simulink model "Copy_of_EmraxEfficiencySimulation"  (R2023b)
settings: Solver=VariableStepAuto  StartTime=0.0  StopTime=2862  MinStep=1e-6  RelTol=1e-3
model workspace (MAT data in the model file):
  surfaceBlockParameters = Simulink.LookupTable
  surfaceBlockParameters.Table = Simulink.lookuptable.Table
  surfaceBlockParameters.Table.Value = [0.86  0.86  0.86  0.86  0.86  0.86  0.86  0.86  0.86  0.86  0.86; 0.86  0.86  0.873462974516  0.88120855107  0.887257540982  0.881274655143  0.875257466166  0.861277049262  0.86  0.86  0.86; 0.86  0.869449686674  0.901077583035  0.940198386719  0.941242897487  0.93026047687  0.938338197526  0.920269194974  0.901654311136  0.876925457275  0.86; 0.86  0.871584749393  0.920465089637  0.946640854986  0.955098186441  0.959157998253  0.952414685218  0.944193761546  0.931829553709  0.909148651806  0.86; 0.86  0.873600000005  0.920099009905  0.957797916669  0.96  0.96  0.955048161402  0.948313069463  0.940179875207  0.910126940639  0.86; 0.86  0.873810561857  0.92068092196  0.957924221415  0.96  0.96  0.954746546712  0.948709551276  0.940686275533  0.907960706815  0.86; 0.86  0.870474457304  0.920710477493  0.954650751967  0.96  0.959091387712  0.953985871947  0.947696813236  0.940596870284  0.905794472991  0.86; 0.86  0.864180163786  0.915794053212  0.947295039135  0.96  0.957068912618  0.952635425118  0.946716594455  0.940428015723  0.903628239166  0.86; 0.86  0.86  0.881189733357  0.926126919259  0.949537413693  0.95356721004  0.95044514073  0.946547739895  0.940259161163  0.900401534397  0.86; 0.86  0.86  0.86  0.89019154205  0.934327668899  0.937067800236  0.945715791697  0.945163394756  0.940090306602  0.909654921019  0.86; 0.86  0.86  0.86  0.86  0.86  0.901026892928  0.936959816894  0.940077714286  0.939615450249  0.908828254349  0.86]
  surfaceBlockParameters.Table.Dimensions = [11 11]
  surfaceBlockParameters.Table.DataType = 'auto'
  surfaceBlockParameters.Table.FieldName = 'Table_Efficiency_Map_Efficiency'
  surfaceBlockParameters.Breakpoints(1) = Simulink.lookuptable.Breakpoint
  surfaceBlockParameters.Breakpoints(1).Value = [0 550 1100 1650 2200 2750 3300 3850 4400 4950 5500]
  surfaceBlockParameters.Breakpoints(1).TunableSizeName = 'N1'
  surfaceBlockParameters.Breakpoints(1).Dimensions = [1 11]
  surfaceBlockParameters.Breakpoints(1).DataType = 'auto'
  surfaceBlockParameters.Breakpoints(1).FieldName = 'BP1_Efficiency_Map_RPM'
  surfaceBlockParameters.Breakpoints(2) = Simulink.lookuptable.Breakpoint
  surfaceBlockParameters.Breakpoints(2).Value = [0 25 50 75 100 125 150 175 200 225 250]
  surfaceBlockParameters.Breakpoints(2).TunableSizeName = 'N2'
  surfaceBlockParameters.Breakpoints(2).Dimensions = [1 11]
  surfaceBlockParameters.Breakpoints(2).DataType = 'auto'
  surfaceBlockParameters.Breakpoints(2).FieldName = 'BP2_Efficiency_Map_Torque'
  surfaceBlockParameters.AllowMultipleInstancesOfTypeToHaveDifferentTableBreakpointSizes = 0
  surfaceBlockParameters.SupportTunableSize = 0
  surfaceBlockParameters.StructTypeInfo = Simulink.lookuptable.StructTypeInfo
  surfaceBlockParameters.StructTypeInfo.Name = 'surfaceBlockParameters_type'
  surfaceBlockParameters.StructTypeInfo.DataScope = 'Auto'
values from neighbouring files (symbols this model uses):
  battery = {}    [init_file.m]
  motor = {}    [init_file.m]
  powertrain = {}    [init_file.m]
libraries: nesl_utility x7, fl_lib x6, batteryecm_lib x1, spsFirstOrderFilterLib x1, mcbcontrolslib x1
settings Model: SimulationMode=accelerator  Creator=benli  LastModifiedBy=benli
settings SolverCC: MaxConsecutiveMinStep=10

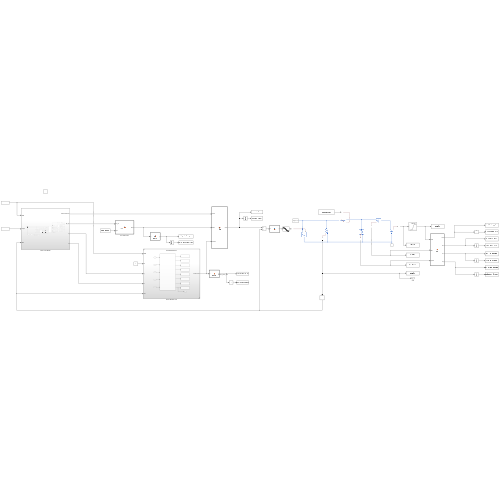
[thumbnail: Simulink's stored preview of the top-level diagram]
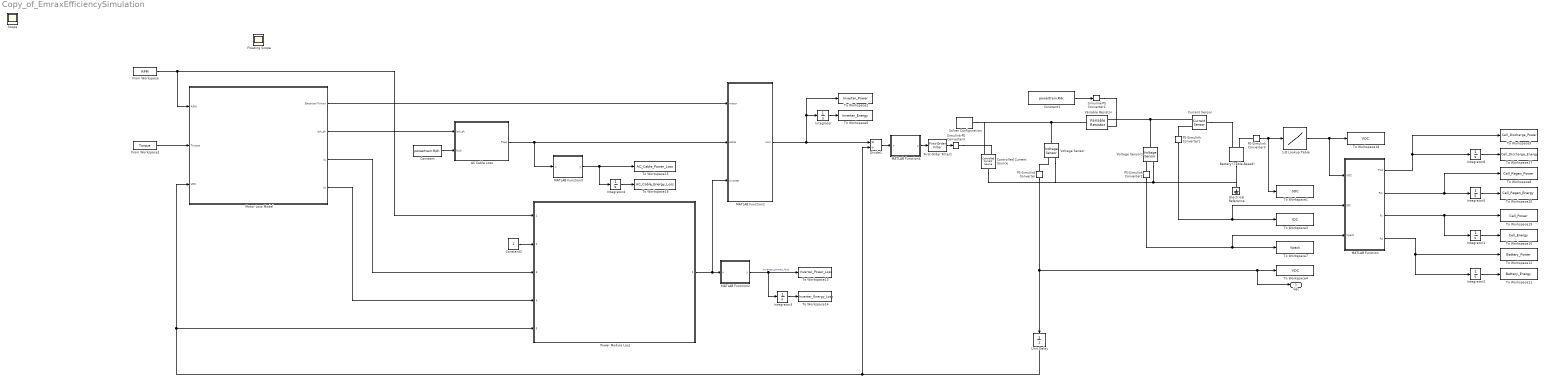
== system Copy_of_EmraxEfficiencySimulation ==
  1-D Lookup Table : Lookup_n-D  NumberOfTableDimensions=1  BreakpointsForDimension1=battery.soc_x_ocv_y(:,1)  Table=battery.soc_x_ocv_y(:,2)*battery.S  InternalRulePriority=Speed  RndMeth=Simplest
  AC Cable Loss : MATLAB Function  TreatAsAtomicUnit=on
  Battery (Table-Based) : batteryecm_lib/Battery (Table-Based)  SOC_vec=battery.soc_x_ocv_y(:,1)  T_dependence=simscape.enum.tablebattery.temperature_dependence.no  prm_dir=simscape.enum.tablebattery.prm_dir.noCurrentDirectionality  T_vec=[278, 293, 313] K  V0_mat=[3.49, 3.5, 3.51; 3.55, 3.57, 3.56; 3.62, 3.63, 3.64; 3.71, 3.71, 3.72; 3.91, 3.93, 3.94; 4.07, 4.08, 4.08; 4.19, 4.19, 4.19] V  V0_vec=battery.soc_x_ocv_y(:,2)*battery.S V  V_range=[0, 700] V  R0_mat=[.0117, .0085, .009; .011, .0085, .009; .0114, .0087, .0092; .0107, .0082, .0088; .0107, .0083, .0091; .0113, .0085, .0089; .0116, .0085, .0089] Ohm  R0_vec=battery.Rdc*ones(1002,1) Ohm  R0_dis_mat=[.0117, .0085, .009; .011, .0085, .009; .0114, .0087, .0092; .0107, .0082, .0088; .0107, .0083, .0091; .0113, .0085, .0089; .0116, .0085, .0089] Ohm  R0_dis_vec=[.0085, .0085, .0087, .0082, .0083, .0085, .0085] Ohm  R0_ch_mat=[.0117, .0085, .009; .011, .0085, .009; .0114, .0087, .0092; .0107, .0082, .0088; .0107, .0083, .0091; .0113, .0085, .0089; .0116, .0085, .0089] Ohm  R0_ch_vec=[.0085, .0085, .0087, .0082, .0083, .0085, .0085] Ohm  AH=battery.Ah*battery.P A*hr  prm_leak=simscape.enum.tablebattery.prm_leak.disabled  Rleak_vec=[8000, 7000, 6000] Ohm  Rleak=7e3 Ohm  extrapolation_option=simscape.enum.extrapolation.linear  SOC_port=simscape.enum.tablebattery.enable.yes  prm_dyn=simscape.enum.tablebattery.prm_dyn.off  R1_mat=[.0109, .0029, .0013; .0069, .0024, .0012; .0047, .0026, .0013; .0034, .0016, .001; .0033, .0023, .0014; .0033, .0018, .0011; .0028, .0017, .0011] Ohm  R1_vec=[.0029, .0024, .0026, .0016, .0023, .0018, .0017] Ohm  tau1_mat=[20, 36, 39; 31, 45, 39; 109, 105, 61; 36, 29, 26; 59, 77, 67; 40, 33, 29; 25, 39, 33] s  tau1_vec=[36, 45, 105, 29, 77, 33, 39] s  R2_mat=[.0109, .0029, .0013; .0069, .0024, .0012; .0047, .0026, .0013; .0034, .0016, .001; .0033, .0023, .0014; .0033, .0018, .0011; .0028, .0017, .0011] Ohm  R2_vec=[.0029, .0024, .0026, .0016, .0023, .0018, .0017] Ohm  tau2_mat=[20, 36, 39; 31, 45, 39; 109, 105, 61; 36, 29, 26; 59, 77, 67; 40, 33, 29; 25, 39, 33] s  tau2_vec=[36, 45, 105, 29, 77, 33, 39] s  R3_mat=[.0109, .0029, .0013; .0069, .0024, .0012; .0047, .0026, .0013; .0034, .0016, .001; .0033, .0023, .0014; .0033, .0018, .0011; .0028, .0017, .0011] Ohm  R3_vec=[.0029, .0024, .0026, .0016, .0023, .0018, .0017] Ohm  tau3_mat=[20, 36, 39; 31, 45, 39; 109, 105, 61; 36, 29, 26; 59, 77, 67; 40, 33, 29; 25, 39, 33] s  tau3_vec=[36, 45, 105, 29, 77, 33, 39] s  R4_mat=[.0109, .0029, .0013; .0069, .0024, .0012; .0047, .0026, .0013; .0034, .0016, .001; .0033, .0023, .0014; .0033, .0018, .0011; .0028, .0017, .0011] Ohm  R4_vec=[.0029, .0024, .0026, .0016, .0023, .0018, .0017] Ohm  tau4_mat=[20, 36, 39; 31, 45, 39; 109, 105, 61; 36, 29, 26; 59, 77, 67; 40, 33, 29; 25, 39, 33] s  tau4_vec=[36, 45, 105, 29, 77, 33, 39] s  R5_mat=[.0109, .0029, .0013; .0069, .0024, .0012; .0047, .0026, .0013; .0034, .0016, .001; .0033, .0023, .0014; .0033, .0018, .0011; .0028, .0017, .0011] Ohm  R5_vec=[.0029, .0024, .0026, .0016, .0023, .0018, .0017] Ohm  tau5_mat=[20, 36, 39; 31, 45, 39; 109, 105, 61; 36, 29, 26; 59, 77, 67; 40, 33, 29; 25, 39, 33] s  tau5_vec=[36, 45, 105, 29, 77, 33, 39] s  prm_fade=simscape.enum.tablebattery.prm_fade.disabled  N0=100  dV0=0  dR0=0  dAH=0  dRleak=0  dR1=0  dR2=0  dR3=0  dR4=0  dR5=0  N0vec=[0, 100, 200, 300]  Tfadevec=[298.15, 323.15] K  dV0vec=[0, 0, 0, 0]  dR0vec=[0, 0, 0, 0]  dAHvec=[0, 0, 0, 0]  dRleakvec=[0, 0, 0, 0]  dR1vec=[0, 0, 0, 0]  dR2vec=[0, 0, 0, 0]  dR3vec=[0, 0, 0, 0]  dR4vec=[0, 0, 0, 0]  dR5vec=[0, 0, 0, 0]  dV0mat=[0, 0; 0, 0; 0, 0; 0, 0]  dR0mat=[0, 0; 0, 0; 0, 0; 0, 0]  dAHmat=[0, 0; 0, 0; 0, 0; 0, 0]  dRleakmat=[0, 0; 0, 0; 0, 0; 0, 0]  dR1mat=[0, 0; 0, 0; 0, 0; 0, 0]  dR2mat=[0, 0; 0, 0; 0, 0; 0, 0]  dR3mat=[0, 0; 0, 0; 0, 0; 0, 0]  dR4mat=[0, 0; 0, 0; 0, 0; 0, 0]  dR5mat=[0, 0; 0, 0; 0, 0; 0, 0]  prm_age_modeling=simscape.enum.tablebattery.prm_age_modeling.equation  storage_dt_age_vec=[0] d  storage_T_age_vec=[273] K  prm_age_OCV=simscape.enum.tablebattery.prm_age_OCV.OCV  OCV_age=0.9  SOC_age=0.6  prm_age_resistance=simscape.enum.tablebattery.prm_age.disabled  OCV_scaling_age_resistance=2.2134e6  OCV_offset_age_resistance=1.632e6  temp_exp_age_resistance=0.515833569 V  t_exp_age_resistance=0.75  T_age_vec_resistance=[273.15, 298.15, 323.15] K  dt_age_vec_resistance=[0, 90, 180, 270] d  dR0_age_vec=[0, 0, 0]  t_meas_dR0_age=100 d  dR0_age_mat=[0, 0, 0; 0, 0, 0; 0, 0, 0; 0, 0, 0]  prm_age_capacity=simscape.enum.tablebattery.prm_age.disabled  OCV_scaling_age_capacity=1.5097e07  OCV_offset_age_capacity=8.3625e06  temp_exp_age_capacity=0.6011 V  t_exp_age_capacity=0.75  T_age_vec_capacity=[273.15, 298.15, 323.15] K  dt_age_vec_capacity=[0, 90, 180, 270] d  dAH_age_vec=[0, 0, 0]  t_meas_dAH_age=100 d  dAH_age_mat=[0, 0, 0; 0, 0, 0; 0, 0, 0; 0, 0, 0]  thermal_port=simscape.enum.thermaleffects.omit  temperature=298.15 K  thermal_mass=100 J/K  i_specify=off  i_priority=None  i=0 A  i_nominal_specify=off  i_nominal_unit=A  i_nominal_value=1  v_specify=off  v_priority=None  v=0 V  v_nominal_specify=off  v_nominal_unit=V  v_nominal_value=1  stateOfCharge_specify=on  stateOfCharge_priority=High  stateOfCharge=0.938  stateOfCharge_nominal_specify=off  stateOfCharge_nominal_unit=1  stateOfCharge_nominal_value=0.95  num_cycles_specify=off  num_cycles_priority=High  num_cycles=0  num_cycles_nominal_specify=off  num_cycles_nominal_unit=1  num_cycles_nominal_value=1  cell_temperature_specify=off  cell_temperature_priority=High  cell_temperature=298.15 K  cell_temperature_nominal_specify=off  cell_temperature_nominal_unit=K  cell_temperature_nominal_value=1
      settings: InternalSimscapePortConfiguration="{\"Bottom\":[],\"Left\":[{\"id\":\"p\",\"label\":\"+\",\"type\":\"foundation.electrical.electrical\"},{\"id\":\"soc\",\"label\":\"SOC\",\"type\":\"output\"}],\"Right\":[{\"id\":\"n\",\"label\":\"-\",\"type\":\"foundation.electrical.electrical\"}],\"Top\":[]}"
      settings: LibrarySourceBlock=|
      | batt_lib/Cells/Battery
      | (Table-Based)
  Constant : Constant  Value=powertrain.Rph
  Constant1 : Constant  Value=powertrain.Rdc
  Constant2 : Constant
  Controlled Current Source : fl_lib/Electrical/Electrical Sources/Controlled Current Source
  Current Sensor : fl_lib/Electrical/Electrical Sensors/Current Sensor
  Divide1 : Product  Inputs=*/
  Electrical Reference : fl_lib/Electrical/Electrical Elements/Electrical Reference
  First-Order Filter1 : spsFirstOrderFilterLib/First-Order Filter  FilterType=Lowpass  Tc=5e-2  Ts=0  Initialize=on  Vac_Init=[0, 0, 60]  Vdc_Init=0  PlotResponse=off  FreqRange="[0,  200,  1]"
  Floating Scope : Scope
      settings: Floating=on
  From Workspace : FromWorkspace  VariableName=RPM  SampleTime=0.05
  From Workspace1 : FromWorkspace  VariableName=Torque  SampleTime=0.05
  Integrator{,1..6} (7 alike) : Integrator
  MATLAB Function : MATLAB Function  TreatAsAtomicUnit=on
  MATLAB Function1 : MATLAB Function  TreatAsAtomicUnit=on
  MATLAB Function2 : MATLAB Function  TreatAsAtomicUnit=on
  MATLAB Function3 : MATLAB Function  TreatAsAtomicUnit=on
  MATLAB Function4 : MATLAB Function  TreatAsAtomicUnit=on
  Motor Loss Model : Subsystem
  PS-Simulink Converter{,1..3} (4 alike) : nesl_utility/PS-Simulink Converter  PhysicalDomain=network_engine_domain  SubClassName=ps_output  LeftPortType=input  RightPortType=output  PseudoPeriodic=off  Frequencies=[]  VectorFormat=inherit  Unit=inherit  AffineConversion=off
  Power Module Loss : Subsystem  ReferencedSubsystem=PowerModuleLoss
  Simulink-PS Converter2 : nesl_utility/Simulink-PS Converter  PhysicalDomain=network_engine_domain  SubClassName=ps_input  LeftPortType=input  RightPortType=output  PseudoPeriodic=off  Frequencies=[]  NoiseDistribution=none  NoiseParameters=[]  Unit=1  AffineConversion=off  FilteringAndDerivatives=provide  SimscapeFilterOrder=1  InputFilterTimeConstant=0.001  UdotUserProvided=0
  Simulink-PS Converter3 : nesl_utility/Simulink-PS Converter  PhysicalDomain=network_engine_domain  SubClassName=ps_input  LeftPortType=input  RightPortType=output  PseudoPeriodic=off  Frequencies=[]  NoiseDistribution=none  NoiseParameters=[]  Unit=1  AffineConversion=off  FilteringAndDerivatives=provide  SimscapeFilterOrder=1  InputFilterTimeConstant=0.001  UdotUserProvided=0
  Solver Configuration : nesl_utility/Solver Configuration  PhysicalDomain=network_engine_domain  SubClassName=solver  LeftPortType=input  RightPortType=generic  Tones=[]  Harmonics=[]  SimulateNoise=off  Profile=off  UseLocalSampling=off  EnableSwitchedLinearOptims=on  FrequencyDomain=off  UseCCode=off  RelTol=0.001  AbsTol=0.001  MinStep=1e-09  ToWorkspace=off  RevertToSquareIcSolve=off  NumHomotopyIterations=100  PhasorMode=off  PhasorModeNumHarmonics=1  ConsistencySolver=NEWTON_XTOL_AFTER_FTOL  IndexReductionMethod=DerivativeReplacement  DoDC=off  ResidualTolerance=1e-09  ConsistencyTolSource=GLOBAL  ConsistencyAbsTol=0.01  ConsistencyRelTol=0.01  ConsistencyTolFactor=0.001  UseLocalSolver=off  LocalSolverChoice=NE_PARTITIONING_ADVANCER  ResolveIndetEquations=on  FunctionEvalNumThread=1  LocalSolverSampleTime=0.0001  DoFixedCost=off  MaxNonlinIter=3  MaxModeIter=2  ComputeImpulses=off  ImpulseIterations=2  LinearAlgebra=auto  LinearAlgebraNumThread=0  EquationFormulation=NE_TIME_EF  DelaysMemoryBudget=1024  AutomaticFiltering=on  FilteringTimeConstant=0.001  PartitionStorageMethod=AS_NEEDED  PartitionMemoryBudget=1024  PartitionMethod=ROBUST  MultibodyUseLocalSolver=off  MultibodyLocalSolverChoice=ODE1  MultibodyLocalSolverSampleTime=0.001
  To Workspace1 : ToWorkspace  VariableName=SOC  SampleTime=-1
  To Workspace10 : ToWorkspace  VariableName=Cell_Energy  SampleTime=-1
  To Workspace11 : ToWorkspace  VariableName=Battery_Energy  SampleTime=-1
  To Workspace12 : ToWorkspace  VariableName=Battery_Power  SampleTime=-1
  To Workspace13 : ToWorkspace  VariableName=Inverter_Power_Loss  SampleTime=-1
  To Workspace14 : ToWorkspace  VariableName=Inverter_Energy_Loss  SampleTime=-1
  To Workspace15 : ToWorkspace  VariableName=AC_Cable_Power_Loss  SampleTime=-1
  To Workspace16 : ToWorkspace  VariableName=AC_Cable_Energy_Loss  SampleTime=-1
  To Workspace17 : ToWorkspace  VariableName=Cell_Discharge_Energy  SampleTime=-1
  To Workspace18 : ToWorkspace  VariableName=VOC  SampleTime=-1
  To Workspace19 : ToWorkspace  VariableName=Cell_Power  SampleTime=-1
  To Workspace2 : ToWorkspace  VariableName=Inverter_Power  SampleTime=-1
  To Workspace20 : ToWorkspace  VariableName=Cell_Regen_Energy  SampleTime=-1
  To Workspace3 : ToWorkspace  VariableName=IDC  SampleTime=-1
  To Workspace4 : ToWorkspace  VariableName=VDC  SampleTime=-1
  To Workspace6 : ToWorkspace  VariableName=Inverter_Energy  SampleTime=-1
  To Workspace7 : ToWorkspace  VariableName=Vpack  SampleTime=-1
  To Workspace8 : ToWorkspace  VariableName=Cell_Regen_Power  SampleTime=-1
  To Workspace9 : ToWorkspace  VariableName=Cell_Discharge_Power  SampleTime=-1
  Unit Delay : UnitDelay  InitialCondition=battery.Voc  SampleTime=-1  HasFrameUpgradeWarning=on
  Variable Resistor : fl_lib/Electrical/Electrical Elements/Variable Resistor  Rmin=1 mOhm  thermalEnable=false  thermal_mass=1 J/K  i_specify=off  i_priority=None  i=0 A  i_nominal_specify=off  i_nominal_unit=A  i_nominal_value=1  v_specify=off  v_priority=None  v=0 V  v_nominal_specify=off  v_nominal_unit=V  v_nominal_value=1  T_specify=off  T_priority=None  T=300 K  T_nominal_specify=off  T_nominal_unit=K  T_nominal_value=1
  Voltage Sensor : fl_lib/Electrical/Electrical Sensors/Voltage Sensor
  Voltage Sensor1 : fl_lib/Electrical/Electrical Sensors/Voltage Sensor
  Vdc : Outport
  Scope : Scope
  wires:
  Constant/1 -> AC Cable Loss/2(Rph)
  Integrator3/1 -> To Workspace14/1
  Power Module Loss/1 -> MATLAB Function1/3(inverter), MATLAB Function2/1(u)
  Motor Loss Model/2(Iph_pk) -> AC Cable Loss/1(Iph_pk)
  From Workspace/1 -> Motor Loss Model/1(RPM), Power Module Loss/1
  MATLAB Function1/1(sum) -> Divide1/1, To Workspace2/1, Integrator/1
  PS-Simulink Converter3/1 -> To Workspace1/1, 1-D Lookup Table/1
  Motor Loss Model/3(Iq) -> Power Module Loss/3
  Unit Delay/1 -> Motor Loss Model/3(VDC), Power Module Loss/5, Divide1/2
  Constant1/1 -> Simulink-PS Converter2/1
  From Workspace1/1 -> Motor Loss Model/2(Torque)
  Motor Loss Model/4(Id) -> Power Module Loss/4
  Motor Loss Model/1(Electrical Power) -> MATLAB Function1/1(motor)
  PS-Simulink Converter1/1 -> To Workspace3/1, MATLAB Function/2(IDC)
  Integrator2/1 -> To Workspace11/1
  Integrator1/1 -> To Workspace10/1
  MATLAB Function3/1(y) -> To Workspace15/1, Integrator4/1
  AC Cable Loss/1(PLac) -> MATLAB Function3/1(u), MATLAB Function1/2(cable)
  Integrator6/1 -> To Workspace17/1
  Constant2/1 -> Power Module Loss/2
  Integrator/1 -> To Workspace6/1
  First-Order Filter1/1 -> Simulink-PS Converter3/1
  Integrator4/1 -> To Workspace16/1
  MATLAB Function/3(Pc) -> To Workspace19/1, Integrator1/1
  MATLAB Function4/1(y) -> First-Order Filter1/1
  1-D Lookup Table/1 -> To Workspace18/1, MATLAB Function/1(VOC)
  MATLAB Function/4(Pp) -> To Workspace12/1, Integrator2/1
  MATLAB Function/2(Pcr) -> To Workspace8/1, Integrator5/1
  MATLAB Function2/1(y) -> To Workspace13/1, Integrator3/1  "inverter_power_loss"
  Integrator5/1 -> To Workspace20/1
  PS-Simulink Converter/1 -> Unit Delay/1, Vdc/1, To Workspace4/1
  PS-Simulink Converter2/1 -> To Workspace7/1, MATLAB Function/3(Vpack)
  MATLAB Function/1(Pcd) -> Integrator6/1, To Workspace9/1
  Divide1/1 -> MATLAB Function4/1(u)
  connections:
  Voltage Sensor1/RConn2 -- Voltage Sensor/RConn2 -- Controlled Current Source/LConn1 -- Battery (Table-Based)/RConn1 -- Electrical Reference/LConn1
  Current Sensor/RConn2 -- Voltage Sensor1/LConn1 -- Variable Resistor/LConn2
  Voltage Sensor/LConn1 -- Controlled Current Source/RConn2 -- Solver Configuration/RConn1 -- Variable Resistor/RConn1
  PS-Simulink Converter3/LConn1 -- Battery (Table-Based)/LConn2
  Current Sensor/LConn1 -- Battery (Table-Based)/LConn1
  Simulink-PS Converter3/RConn1 -- Controlled Current Source/RConn1
  Current Sensor/RConn1 -- PS-Simulink Converter1/LConn1
  Simulink-PS Converter2/RConn1 -- Variable Resistor/LConn1
  PS-Simulink Converter/LConn1 -- Voltage Sensor/RConn1
  PS-Simulink Converter2/LConn1 -- Voltage Sensor1/RConn1

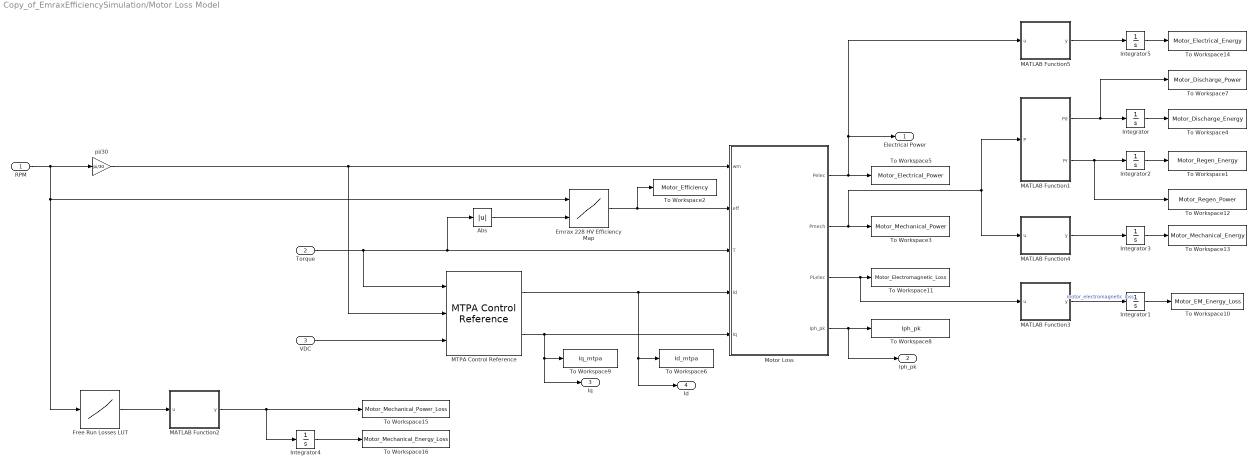
== system Copy_of_EmraxEfficiencySimulation/Motor Loss Model ==
  RPM : Inport
  Torque : Inport  Port=2
  VDC : Inport  Port=3
  Abs : Abs  SaturateOnIntegerOverflow=off
  Emrax 228 HV Efficiency Map : Lookup_n-D  DataSpecification=Lookup table object  LookupTableObject=surfaceBlockParameters  BreakpointsForDimension1=[1:3]  BreakpointsForDimension2=[1:3]  ExtrapMethod=Clip  InternalRulePriority=Speed  RndMeth=Simplest
      settings: AttributesFormatString=Extrapolation=%<ExtrapMethod>  InputPortMap=u0,u1
  Free Run Losses LUT : Lookup_n-D  NumberOfTableDimensions=1  BreakpointsForDimension1=motor.RPM_x_Power_y(:, 1)  Table=motor.RPM_x_Power_y(:, 2)  InternalRulePriority=Speed  RndMeth=Simplest
  Integrator{,1..5} (6 alike) : Integrator
  MATLAB Function1 : MATLAB Function  TreatAsAtomicUnit=on
  MATLAB Function2 : MATLAB Function  TreatAsAtomicUnit=on
  MATLAB Function3 : MATLAB Function  TreatAsAtomicUnit=on
  MATLAB Function4 : MATLAB Function  TreatAsAtomicUnit=on
  MATLAB Function5 : MATLAB Function  TreatAsAtomicUnit=on
  MTPA Control Reference : mcbcontrolslib/MTPA Control Reference  VariantSelect=Interior PMSM  polePairs=motor.Pp  Rs=motor.Rw  Ld=motor.Ld  Lq=motor.Lq  FluxPM=motor.Lambda_m  ilimit=motor.I_lim  Vdc_input_select=Input port  V_dc=500  Units=SI Units  N_base=4107  I_base=19.3  T_base=1  V_base=24/sqrt(3)  N_base_disp=3182  MTPAiterator=on  iterCount=10
      settings: LibrarySourceBlock=mcblib/Controls/Control Reference/MTPA Control Reference
  Motor Loss : MATLAB Function  TreatAsAtomicUnit=on
  To Workspace1 : ToWorkspace  VariableName=Motor_Regen_Energy  SampleTime=-1
  To Workspace10 : ToWorkspace  VariableName=Motor_EM_Energy_Loss  SampleTime=-1
  To Workspace11 : ToWorkspace  VariableName=Motor_Electromagnetic_Loss  SampleTime=-1
  To Workspace12 : ToWorkspace  VariableName=Motor_Regen_Power  SampleTime=-1
  To Workspace13 : ToWorkspace  VariableName=Motor_Mechanical_Energy  SampleTime=-1
  To Workspace14 : ToWorkspace  VariableName=Motor_Electrical_Energy  SampleTime=-1
  To Workspace15 : ToWorkspace  VariableName=Motor_Mechanical_Power_Loss  SampleTime=-1
  To Workspace16 : ToWorkspace  VariableName=Motor_Mechanical_Energy_Loss  SampleTime=-1
  To Workspace2 : ToWorkspace  VariableName=Motor_Efficiency  SampleTime=-1
  To Workspace3 : ToWorkspace  VariableName=Motor_Mechanical_Power  SampleTime=-1
  To Workspace4 : ToWorkspace  VariableName=Motor_Discharge_Energy  SampleTime=-1
  To Workspace5 : ToWorkspace  VariableName=Motor_Electrical_Power  SampleTime=-1
  To Workspace6 : ToWorkspace  VariableName=Id_mtpa  SampleTime=-1
  To Workspace7 : ToWorkspace  VariableName=Motor_Discharge_Power  SampleTime=-1
  To Workspace8 : ToWorkspace  VariableName=Iph_pk  SampleTime=-1
  To Workspace9 : ToWorkspace  VariableName=Iq_mtpa  SampleTime=-1
  pi/30 : Gain  Gain=pi/30
  Electrical Power : Outport
  Iph_pk : Outport  Port=2
  Iq : Outport  Port=3  OutDataTypeStr=double
  Id : Outport  Port=4  OutDataTypeStr=double
  wires:
  Torque/1 -> MTPA Control Reference/1, Motor Loss/3(T), Abs/1
  pi/30/1 -> MTPA Control Reference/2, Motor Loss/1(wm)
  VDC/1 -> MTPA Control Reference/3
  MATLAB Function5/1(y) -> Integrator5/1
  MATLAB Function4/1(y) -> Integrator3/1
  MATLAB Function1/1(Pd) -> To Workspace7/1, Integrator/1
  Motor Loss/2(Pmech) -> To Workspace3/1, MATLAB Function4/1(u), MATLAB Function1/1(P)
  Integrator5/1 -> To Workspace14/1
  Integrator/1 -> To Workspace4/1
  Integrator3/1 -> To Workspace13/1
  Motor Loss/1(Pelec) -> Electrical Power/1, MATLAB Function5/1(u), To Workspace5/1
  MATLAB Function1/2(Pr) -> Integrator2/1, To Workspace12/1
  Integrator2/1 -> To Workspace1/1
  MATLAB Function3/1(y) -> Integrator1/1  "motor_electromagnetic_loss"
  Integrator1/1 -> To Workspace10/1
  MATLAB Function2/1(y) -> To Workspace15/1, Integrator4/1
  Motor Loss/3(PLelec) -> To Workspace11/1, MATLAB Function3/1(u)
  Free Run Losses LUT/1 -> MATLAB Function2/1(u)
  Integrator4/1 -> To Workspace16/1
  Emrax 228 HV Efficiency Map/1 -> To Workspace2/1, Motor Loss/2(eff)
  RPM/1 -> pi/30/1, Emrax 228 HV Efficiency Map/1, Free Run Losses LUT/1
  MTPA Control Reference/1 -> Id/1, To Workspace6/1, Motor Loss/4(Id)
  MTPA Control Reference/2 -> Motor Loss/5(Iq), Iq/1, To Workspace9/1
  Abs/1 -> Emrax 228 HV Efficiency Map/2
  Motor Loss/4(Iph_pk) -> To Workspace8/1, Iph_pk/1

== matlab function Copy_of_EmraxEfficiencySimulation/Motor Loss Model/MATLAB Function1 ==
  data: P input; Pd output; Pr output
function [Pd, Pr] = power(P)
    if isnan(P)
        Pd = 0;
        Pr = 0;
    elseif P>0
        Pd = P;
        Pr = 0;
    else
        Pd = 0;
        Pr = -P;
    end
end

== matlab function Copy_of_EmraxEfficiencySimulation/Motor Loss Model/MATLAB Function5 ==
  data: u input; y output
function y = power(u)
    if isnan(u)
        y = 0;
    else
        y = u;
    end
end

== matlab function Copy_of_EmraxEfficiencySimulation/MATLAB Function ==
  data: Pcd output; VOC input; IDC input; Pcr output; Pc output; Vpack input; Pp output
function [Pcd, Pcr, Pc, Pp] = fcn(VOC, IDC, Vpack)
    if IDC>0
        Pcr = 0;
        Pcd = IDC * VOC;
    else
        Pcr = -IDC * VOC;
        Pcd = 0;
    end
    Pc = IDC * VOC;
    Pp = IDC * Vpack;
end

== matlab function Copy_of_EmraxEfficiencySimulation/AC Cable Loss ==
  data: PLac output; Iph_pk input; Rph input
function PLac = ACCableLoss(Iph_pk, Rph)

    PLac = 1.5 * (Iph_pk)^2 * Rph;

end

== matlab function Copy_of_EmraxEfficiencySimulation/Motor Loss Model/Motor Loss ==
  data: Pelec output; Pmech output; PLelec output; wm input; eff input; T input; Id input double size=1; Iq input double size=1; Iph_pk output
function [Pelec, Pmech, PLelec, Iph_pk] = MotorLoss(wm, eff, T, Id, Iq)
    Pelec = wm * T;
    if Pelec >= 0
        Pmech = Pelec * (eff);
    else
        Pmech = Pelec * (1/eff);
    end
    PLelec = Pelec - Pmech;
    Iph_pk = (Id^2 + Iq^2)^0.5;
end

== matlab function Copy_of_EmraxEfficiencySimulation/MATLAB Function1 ==
  data: motor input; sum output; cable input; inverter input
function sum = Ptotal(motor, cable, inverter)
sum = motor + cable + inverter;
    if isnan(sum)
        sum = 0;
    end
end

== matlab function Copy_of_EmraxEfficiencySimulation/Motor Loss Model/MATLAB Function2 ==
  data: u input; y output
function y = power(u)
    if isnan(u)
        y = 0;
    else
        y = u;
    end
end

== matlab function Copy_of_EmraxEfficiencySimulation/MATLAB Function2 ==
  data: u input; y output
function y = power(u)
    if isnan(u)
        y = 0;
    else
        y = u;
    end
end

== matlab function Copy_of_EmraxEfficiencySimulation/MATLAB Function3 ==
  data: u input; y output
function y = power(u)
    if isnan(u)
        y = 0;
    else
        y = u;
    end
end

== matlab function Copy_of_EmraxEfficiencySimulation/Motor Loss Model/MATLAB Function3 ==
  data: u input; y output
function y = power(u)
    if isnan(u)
        y = 0;
    else
        y = u;
    end
end

== matlab function Copy_of_EmraxEfficiencySimulation/MATLAB Function4 ==
  data: u input; y output
function y = current(u)
    if isnan(u)
        y = 0;
    else
        y = u;
    end
end

== matlab function Copy_of_EmraxEfficiencySimulation/Motor Loss Model/MATLAB Function4 ==
  data: u input; y output
function y = power(u)
    if isnan(u)
        y = 0;
    else
        y = u;
    end
end
